simulink model "arabaStm"  (R2023b)
settings: Solver=FixedStepAuto  StartTime=0.0  StopTime=45  RelTol=1e-3  EnableMultiTasking=on
undefined symbols (not defined in the file): PosCtrlSpeedLimit
libraries: stm32f4xxblockslib x11, stm32blockslib x4, mcbpositiondecoderlib x3, simulink x1, lidarlib x1, slpidlib x1, mcbcontrolslib x1, slrealtimeiplib x1
settings Model: Creator=The MathWorks, Inc.  LastModifiedBy=yigit
settings OptimizationCC: EnhancedBackFolding=on  PassReuseOutputArgsAs=Individual arguments  ZeroExternalMemoryAtStartup=off  ZeroInternalMemoryAtStartup=off  MaxStackSize=64  OptimizeBlockOrder=speed  DifferentSizesBufferReuse=on  OptimizationCustomize=off  EfficientTunableParamExpr=on
settings DebuggingCC: ParameterTunabilityLossMsg=error  UnconnectedInputMsg=warning  UnconnectedOutputMsg=warning  UnconnectedLineMsg=warning  SubsystemReferenceDiagnosticForUnitTest=warning
settings HardwareCC: ProdBitPerPointer=32  ProdBitPerSizeT=32  ProdBitPerPtrDiffT=32  ProdLargestAtomicInteger=Long  ProdLargestAtomicFloat=Double  ProdWordSize=32  ProdLongLongMode=on  ProdHWDeviceType=ARM Compatible->ARM Cortex
settings ModelReferenceCC: EnableRefExpFcnMdlSchedulingChecks=on
settings SFSimCC: MATLABDynamicMemAlloc=off
settings RTWCC: Description=Embedded Coder  SystemTargetFile=ert.tlc  HardwareBoard=STM32F4xx Based  TemplateMakefile=ert_default_tmf  Toolchain=GNU Tools for ARM Embedded Processors  DLArmComputeVersion=19.05
settings CodeAppCC: ForceParamTrailComments=on  IgnoreCustomStorageClasses=off  OperatorAnnotations=on  SimulinkDataObjDesc=on  SFDataObjDesc=on  InsertBlockDesc=on
settings ERTTargetCC: CodeReplacementLibrary=ARM Cortex-M  ExtModeTransport=3  ExtModeStaticAlloc=on  ExtModeStaticAllocSize=8000  ExtModeMexFile=ext_xcp  ExtModeIntrfLevel=Level2 - Open

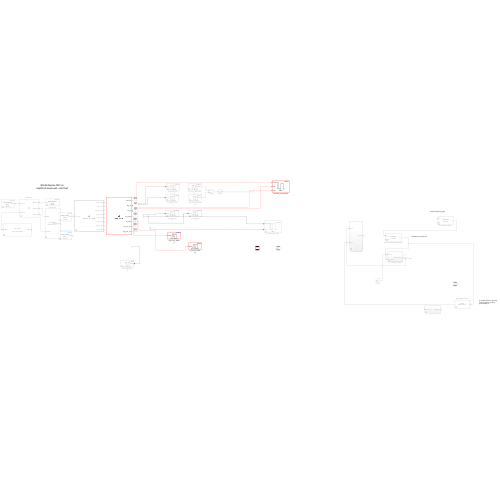
[thumbnail: Simulink's stored preview of the top-level diagram]
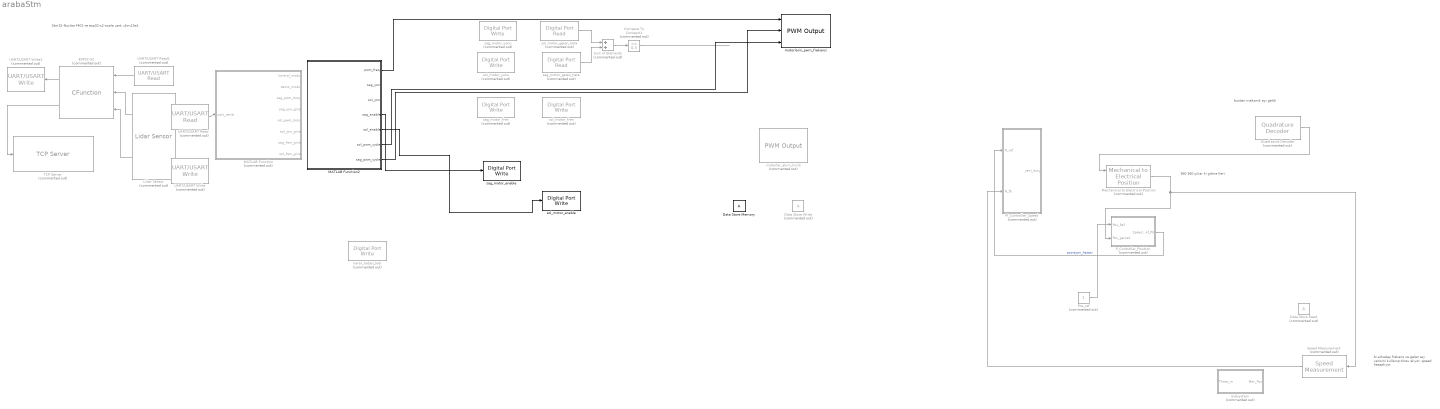
== system arabaStm ==
  note: bı arkadaş frekans ve gelen açı verisini kullanıp türev alıyor. speed hesaplıyor
  note: 360 360 çıkar ki gitme ileri.
  note: burdan mekanik açı geldi
  note: Stm32-Nucleo f401-re
      | esp32-s2-soala uart, uhm15a1
  Compare To Constant1 : simulink/Logic and Bit Operations/Compare To Constant  Commented=on  relop=>=  const=0.5  OutDataTypeStr=boolean
  Data Store Memory : DataStoreMemory  WriteAfterWriteMsg=warning  ShowAdditionalParam=off  OutDataTypeStr=single
  Data Store Read : DataStoreRead  Commented=on  IndexOptions=Index vector (dialog)  Indices=1  OutputSizes=1
  Data Store Write : DataStoreWrite  Commented=on  IndexOptions=Index vector (dialog)  Indices=1  OutputSizes=1
  ESP32-S2 : CFunction  Commented=on  StartCode=|
      | function [motor1_speed, motor2_speed, duration] = simulateESP32Block()
      | %#codegen
      | 
      | % Define the function to simulate ESP32 behavior
      | coder.inline('never');
      | coder.extrinsic('rand');
      | 
      | % Initialize the motor control data structure
      | data.motor1_speed = uint8(0);
      | data.motor2_speed = uint8(0);
      | data.duration = uint8(0);
      | 
      | % Call the function to simulate ESP32 behavior
      | data = simulateESP32();
      | 
      | % Extract the fields from the structure
      | motor1_speed = data.motor1_speed;
      | motor2_speed = data.motor2_speed;
      | duration = data.duration;
      | 
      | end
      | 
      | % Define the function simulateESP32 within the same file
      | function data = simulateESP32()
      | % Simulate receiving motor control data
      | 
      | % Initialize random seed
      | coder.extrinsic('rng');
      | rng('shuffle');
      | 
      | % Create a structure for motor control data
      | data.motor1_speed = uint8(rand() * 255);
      | data.motor2_speed = uint8(rand() * 255);
      | data.duration = uint8(rand() * 60);
      | 
      | end
  Lidar Sensor : lidarlib/Lidar Sensor  Commented=on  SensorIndex=1  UpdateRate=0.1  SensorPosition=[0 0.2 0]  SensorOrientation=[0 0 0]  ActorProfilesVariableName=disable  HostID=1  MaxRange=120  AzimuthLimits=[-180 180]  AzimuthResolution=0.16  UseCustomElevationAngles=off  ElevationAngles=[-25 -15.6 -11.3 -8.8:0.9:-4 -4:0.32:1.6 3.3 4.6 7 10.3 15]  ElevationLimits=[-20 20]  ElevationResolution=1.25  HasNoise=on  RangeAccuracy=0.002  FogVisibility=1000  Rainrate=0  OutputIntensity=off  OutputClusters=off
  MATLAB Function : MATLAB Function  Commented=on  TreatAsAtomicUnit=on
  MATLAB Function2 : MATLAB Function  TreatAsAtomicUnit=on
  Mechanical to Electrical Position : mcbpositiondecoderlib/Mechanical to Electrical Position  Commented=on  PolePairsInputType=Specify via dialog  NrPP=4  selectedRange=Per unit  MechOfstInputType=Input port  mechOffsetIn=0  maxAngleIn=1  InputDataType=single  VariantSelect=floating-point
      settings: LibrarySourceBlock=mcblib/Sensor Decoders/Mechanical to Electrical Position
  PI_Controller_Speed : Subsystem  Commented=on
  P_Controller_Position : Subsystem  Commented=on
  Pos_ref : Constant  Commented=on  OutDataTypeStr=single  SampleTime=-1
  Quadrature Decoder : mcbpositiondecoderlib/Quadrature Decoder  Commented=on  EncoderSlitsPerRevolution=1000  EncoderCountsPerSlit=4  CounterSize=16 bits  ExternalIndexCount=on  PositionUnit=Radians  PositionDataType=single  ParameterInputType=off  CountsPerRevInverseDataType=single
      settings: LibrarySourceBlock=mcblib/Sensor Decoders/Quadrature Decoder
  Speed Measurement : mcbpositiondecoderlib/Speed Measurement  Commented=on  PositionUnit=Radians  PositionScalingDatatype=uint32  SpeedCalculationMode=Maximum application speed  SampleTimeAsync=100e-6  MaximumApplicationSpeed=1000  SpeedResolution=5e-6  DelayLength=299  MaximumMeasurableSpeed=1000  MeasurableSpeedResolution=4.6566e-07  SpeedUnit=RPM  PerUnitSpeed=1000  SpeedDataType=single
      settings: LibrarySourceBlock=mcblib/Sensor Decoders/Speed Measurement
  Subsystem : Subsystem  Commented=on
  Sum of Elements : Sum  Commented=on  OutMin=2
  TCP Server : slrealtimeiplib/TCP Server  Priority=-1  Commented=on  useHostTargetConn=off  serverAddress=192.168.1.95  serverPort=8001
  UART/USART Read : stm32blockslib/UART//USART Read  Priority=2  Commented=on  UARTModule=USART6  DataType=uint8  DataLength=8  BlockingMode=off  BlockingTimeout=0.1  OutputLength=off  OutputStatus=off  SampleTime=-1
      settings: LibrarySourceBlock=stm32f4xxblockslib/UART//USART Read
  UART/USART Read1 : stm32blockslib/UART//USART Read  Priority=2  Commented=on  UARTModule=USART2  DataType=uint8  DataLength=8  BlockingMode=off  BlockingTimeout=0.1  OutputLength=off  OutputStatus=off  SampleTime=-1
      settings: LibrarySourceBlock=stm32f4xxblockslib/UART//USART Read
  UART/USART Write : stm32blockslib/UART//USART Write  Priority=1  Commented=on  UARTModule=USART6  LengthOfDataToSend=off  BlockingMode=off  BlockingTimeout=0.1  OutputStatus=off
      settings: LibrarySourceBlock=stm32f4xxblockslib/UART//USART Write
  UART/USART Write1 : stm32blockslib/UART//USART Write  Priority=1  Commented=on  UARTModule=USART1  LengthOfDataToSend=off  BlockingMode=off  BlockingTimeout=0.1  OutputStatus=off
      settings: LibrarySourceBlock=stm32f4xxblockslib/UART//USART Write
  karar_hatasi_ledi : stm32f4xxblockslib/Digital Port Write  Commented=on  PortName=GPIOB  PinNumber=[0]  ReadOperation=off  IOAsArray=on  EnableSimPort=off
      settings: AttributesFormatString=%<PinNumber>
  motorlar_akim_limiti : stm32f4xxblockslib/PWM Output  Commented=on  TimerModule=TIM3  DutycycleUnits=Percentage  EnableChannel1=on  EnableChannel2=off  EnableChannel3=off  EnableChannel4=off  EnableCounterInput=off  EnableMainOutputInput=off  EnableFrequencyInput=on  SetRCAfterCE=off  OutputDirection=off  OutputMainOutputEnableStatus=off  SampleTime=0.1  EnableSimPort=off  EnableUpdateEvent=off  EnableCaptureCompare1Event=off  EnableCaptureCompare2Event=off  EnableCaptureCompare3Event=off  EnableCaptureCompare4Event=off  EnableTriggerEvent=off  EnableBreakEvent=on  ProcessorFamily=STM32F4  hoistedMaskSrc=ECSoC/ECSimCodegen/PWM Output
  motorlarin_pwm_frekansi : stm32f4xxblockslib/PWM Output  TimerModule=TIM3  DutycycleUnits=Percentage  EnableChannel1=on  EnableChannel2=on  EnableChannel3=off  EnableChannel4=off  EnableCounterInput=off  EnableMainOutputInput=off  EnableFrequencyInput=on  SetRCAfterCE=off  OutputDirection=off  OutputMainOutputEnableStatus=off  SampleTime=0.1  EnableSimPort=off  EnableUpdateEvent=off  EnableCaptureCompare1Event=off  EnableCaptureCompare2Event=off  EnableCaptureCompare3Event=off  EnableCaptureCompare4Event=off  EnableTriggerEvent=off  EnableBreakEvent=on  ProcessorFamily=STM32F4  hoistedMaskSrc=ECSoC/ECSimCodegen/PWM Output
  sag_motor_enable : stm32f4xxblockslib/Digital Port Write  PortName=GPIOA  PinNumber=[7]  ReadOperation=off  IOAsArray=on  EnableSimPort=off
      settings: AttributesFormatString=%<PinNumber>
  sag_motor_fren : stm32f4xxblockslib/Digital Port Write  Commented=on  PortName=GPIOB  PinNumber=[1]  ReadOperation=off  IOAsArray=on  EnableSimPort=off
      settings: AttributesFormatString=%<PinNumber>
  sag_motor_gelen_hata : stm32f4xxblockslib/Digital Port Read  Commented=on  PortName=GPIOA  PinNumber=[10]  ReadOperation=on  IOAsArray=on  SampleTime=-1  EnableSimPort=off
      settings: AttributesFormatString=%<PinNumber>
  sag_motor_yonu : stm32f4xxblockslib/Digital Port Write  Commented=on  PortName=GPIOA  PinNumber=[0]  ReadOperation=off  IOAsArray=on  EnableSimPort=off
      settings: AttributesFormatString=%<PinNumber>
  sol_motor_enable : stm32f4xxblockslib/Digital Port Write  PortName=GPIOA  PinNumber=[10]  ReadOperation=off  IOAsArray=on  EnableSimPort=off
      settings: AttributesFormatString=%<PinNumber>
  sol_motor_fren : stm32f4xxblockslib/Digital Port Write  Commented=on  PortName=GPIOB  PinNumber=[2]  ReadOperation=off  IOAsArray=on  EnableSimPort=off
      settings: AttributesFormatString=%<PinNumber>
  sol_motor_gelen_hata : stm32f4xxblockslib/Digital Port Read  Commented=on  PortName=GPIOA  PinNumber=[11]  ReadOperation=on  IOAsArray=on  SampleTime=-1  EnableSimPort=off
      settings: AttributesFormatString=%<PinNumber>
  sol_motor_yonu : stm32f4xxblockslib/Digital Port Write  Commented=on  PortName=GPIOA  PinNumber=[1]  ReadOperation=off  IOAsArray=on  EnableSimPort=off
      settings: AttributesFormatString=%<PinNumber>
  wires:
  UART/USART Read/1 -> MATLAB Function/1(uart_verisi)
  UART/USART Read1/1 -> ESP32-S2/1
  ESP32-S2/1 -> UART/USART Write1/1
  ESP32-S2/2 -> TCP Server/1
  Lidar Sensor/1 -> ESP32-S2/2
  Lidar Sensor/2 -> ESP32-S2/3
  ? -> sag_motor_yonu/1
  Sum of Elements/1 -> Compare To Constant1/1
  Compare To Constant1/1 -> ?
  ? -> sol_motor_yonu/1
  ? -> sol_motor_fren/1
  ? -> sag_motor_fren/1
  ? -> karar_hatasi_ledi/1
  sol_motor_gelen_hata/1 -> Sum of Elements/1
  sag_motor_gelen_hata/1 -> Sum of Elements/2
  MATLAB Function2/1(pwm_freq) -> motorlarin_pwm_frekansi/1
  MATLAB Function2/7(sag_pwm_cycle) -> motorlarin_pwm_frekansi/2
  MATLAB Function2/6(sol_pwm_cycle) -> motorlarin_pwm_frekansi/3
  ? -> motorlar_akim_limiti/1
  ? -> motorlar_akim_limiti/2
  MATLAB Function2/4(sag_enable) -> sag_motor_enable/1
  MATLAB Function2/5(sol_enable) -> sol_motor_enable/1
  Quadrature Decoder/1 -> Mechanical to Electrical Position/1
  Mechanical to Electrical Position/1 -> P_Controller_Position/2(Pos_gercek), Speed Measurement/1
  P_Controller_Position/1(Speed_Ref_PU) -> PI_Controller_Speed/1(N_ref)  "pozisyon_hatasi"
  Speed Measurement/1 -> PI_Controller_Speed/2(N_fb)
  Pos_ref/1 -> P_Controller_Position/1(Pos_Ref)

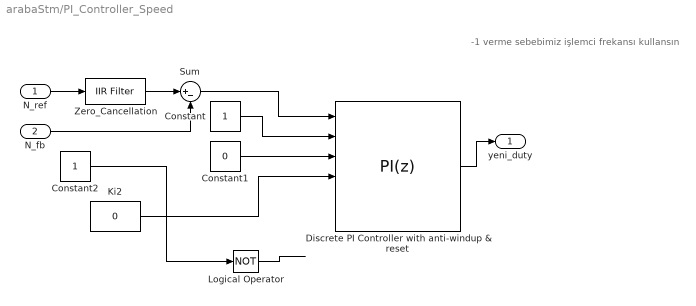
== system arabaStm/PI_Controller_Speed ==
  note: -1 verme sebebimiz işlemci frekansı kullansın
  N_ref : Inport
  N_fb : Inport  Port=2
  Constant : Constant
  Constant1 : Constant  Value=0
  Constant2 : Constant
  Discrete PI Controller with anti-windup & reset : slpidlib/PID Controller  Controller=PI  Form=Parallel  TimeDomain=Discrete-time  UseExternalTs=off  SampleTime=-1  IntegratorMethod=Forward Euler  FilterMethod=Forward Euler  ControllerParametersSource=external  P=1  I=1  UseKiTs=on  D=0  N=100  UseFilter=on  TunerSelectOption=Transfer Function Based (PID Tuner App)  InitialConditionSource=external  InitialConditionForIntegrator=0  InitialConditionForFilter=0  DifferentiatorICPrevScaledInput=0  ExternalReset=none  TrackingMode=off  Kt=1  LimitOutput=on  SatLimitsSource=external  UpperSaturationLimit=1  LowerSaturationLimit=-1  LinearizeAsGain=on  AntiWindupMode=none  Kb=1  LimitIntegrator=off  UpperIntegratorSaturationLimit=inf  LowerIntegratorSaturationLimit=-inf  RndMeth=Simplest  POutMin=[]  POutMax=[]  IOutMin=[]  IOutMax=[]  DOutMin=[]  DOutMax=[]  NOutMin=[]  NOutMax=[]  SumOutMin=[]  SumOutMax=[]  SaturationOutDataTypeStr=Inherit: Inherit via back propagation  SaturationOutMin=[]  SaturationOutMax=[]  PParamMin=[]  PParamMax=[]  IParamMin=[]  IParamMax=[]  DParamMin=[]  DParamMax=[]  NParamMin=[]  NParamMax=[]  KbParamMin=[]  KbParamMax=[]  KtParamMin=[]  KtParamMax=[]  KbOutMin=[]  KbOutMax=[]  KtOutMin=[]  KtOutMax=[]  IntegratorOutMin=[]  IntegratorOutMax=[]  FilterOutMin=[]  FilterOutMax=[]  SumI1OutMin=[]  SumI1OutMax=[]  SumI2OutMin=[]  SumI2OutMax=[]  SumI3OutMin=[]  SumI3OutMax=[]  SumI4OutMin=[]  SumI4OutMax=[]  SumDOutMin=[]  SumDOutMax=[]  DifferentiatorOutMin=[]  DifferentiatorOutMax=[]  FilterDiffOutCoefMin=[]  FilterDiffOutCoefMax=[]  ReciprocalOutMin=[]  ReciprocalOutMax=[]  SumDenOutMin=[]  SumDenOutMax=[]  SumNumOutMin=[]  SumNumOutMax=[]  DivideOutMin=[]  DivideOutMax=[]  UdiffTsProdOutMin=[]  UdiffTsProdOutMax=[]  NTsProdOutMin=[]  NTsProdOutMax=[]  UintegralTsProdOutMin=[]  UintegralTsProdOutMax=[]  UngainTsProdOutMin=[]  UngainTsProdOutMax=[]  ClampingZeroOutDataTypeStr=Inherit: Inherit via back propagation  ClampingZeroOutMin=[]  ClampingZeroOutMax=[]  FilterDenConstantOutDataTypeStr=Inherit: Inherit via back propagation  FilterDenConstantOutMin=[]  FilterDenConstantOutMax=[]  PCopyOutDataTypeStr=Inherit: Inherit via back propagation  PCopyOutMin=[]  PCopyOutMax=[]  NCopyOutDataTypeStr=Inherit: Inherit via back propagation  NCopyOutMin=[]  NCopyOutMax=[]  IntegratorContinuousStateAttributes=''  IntegratorStateMustResolveToSignalObject=off  IntegratorRTWStateStorageClass=Auto  FilterContinuousStateAttributes=''  FilterStateMustResolveToSignalObject=off  FilterRTWStateStorageClass=Auto  ParallelPVariant=ExternalParameters  IdealPVariant=Disabled  IVariant=ExternalParameters  DVariant=Disabled  IntegratorVariant=Discrete  SatVariant=External  AWVariant=Passthrough  PCopyVariant=Disabled  TRVariant=Disabled  FdbkBlocksVariant=Forward  IdealPFdbkVariant=Disabled  SatFdbkVariant=Disabled  DerivativeFilterVariant=Disabled  NVariant=Disabled  NCopyVariant=Disabled_SignalSpec  FilterICVariant=Disabled  IntegratorICVariant=ExternalICs  ExternalResetVariant=Disabled  TRSumVariant=Passthrough  SumFdbkVariant=Disabled  SumVariant=Sum_PI  TsampFilterVariant=InternalTs  TsampNgainVariant=Passthrough  TsampIntegralVariant=Disabled_SignalSpec  ExternalSaturationOutDataTypeStr=Inherit: Same as second input
      settings: LibrarySourceBlock=mcbcontrolslib/PI Controller
  Ki2 : Constant  Value=0  OutDataTypeStr=single  SampleTime=-1
  Logical Operator : Logic  Operator=NOT  IconShape=distinctive  AllPortsSameDT=off  OutDataTypeStr=boolean
  Sum : Sum  Inputs=|+-  RndMeth=Round
  Zero_Cancellation : mcbcontrolslib/IIR Filter  VariantControl=Low Pass Filter  VariantSelect=Low-pass  Filter_constant=0.01  advancedSettings=off  Ts=50e-6  cutOff_freq=32.1525
  yeni_duty : Outport  VectorParamsAs1DForOutWhenUnconnected=off
  wires:
  Discrete PI Controller with anti-windup & reset/1 -> yeni_duty/1
  Constant1/1 -> Discrete PI Controller with anti-windup & reset/3
  Constant/1 -> Discrete PI Controller with anti-windup & reset/2
  N_fb/1 -> Sum/2
  N_ref/1 -> Zero_Cancellation/1
  Logical Operator/1 -> ?
  Ki2/1 -> Discrete PI Controller with anti-windup & reset/4
  Sum/1 -> Discrete PI Controller with anti-windup & reset/1
  Constant2/1 -> Logical Operator/1
  Zero_Cancellation/1 -> Sum/1

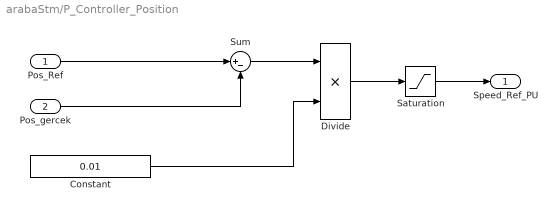
== system arabaStm/P_Controller_Position ==
  Pos_Ref : Inport
  Pos_gercek : Inport  Port=2
  Constant : Constant  Value=0.01  OutDataTypeStr=single  SampleTime=-1
  Divide : Product  Inputs=**  OutDataTypeStr=single  RndMeth=Simplest
  Saturation : Saturate  UpperLimit=PosCtrlSpeedLimit  LowerLimit=-PosCtrlSpeedLimit
  Sum : Sum  Inputs=|+-  OutDataTypeStr=Inherit: Same as first input
  Speed_Ref_PU : Outport
  wires:
  Constant/1 -> Divide/2
  Saturation/1 -> Speed_Ref_PU/1
  Divide/1 -> Saturation/1
  Pos_Ref/1 -> Sum/1
  Pos_gercek/1 -> Sum/2
  Sum/1 -> Divide/1

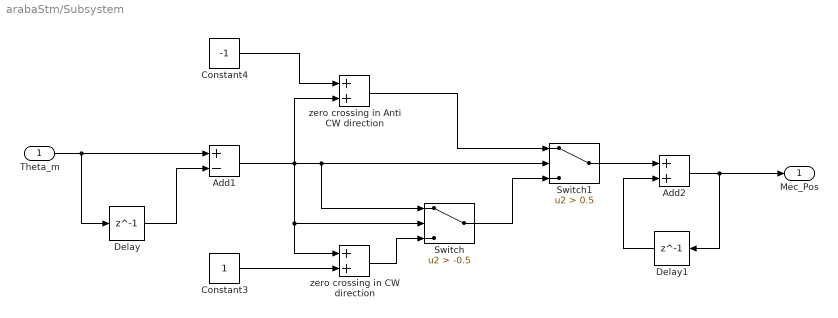
== system arabaStm/Subsystem ==
  Theta_m : Inport
  Add1 : Sum  Inputs=+-
  Add2 : Sum
  Constant3 : Constant  OutDataTypeStr=dataType
  Constant4 : Constant  Value=-1  OutDataTypeStr=dataType
  Delay : Delay  DelayLength=1
  Delay1 : Delay  DelayLength=1
  Switch : Switch  Criteria=u2 > Threshold  Threshold=-0.5  SaturateOnIntegerOverflow=off  InputSameDT=off
  Switch1 : Switch  Criteria=u2 > Threshold  Threshold=0.5  SaturateOnIntegerOverflow=off  InputSameDT=off
  zero crossing in Anti CW direction : Sum
  zero crossing in CW direction : Sum
  Mec_Pos : Outport
  wires:
  Theta_m/1 -> Delay/1, Add1/1
  Switch1/1 -> Add2/1
  Delay/1 -> Add1/2
  Add1/1 -> zero crossing in Anti CW direction/2, zero crossing in CW direction/1, Switch/2, Switch/1, Switch1/2
  Switch/1 -> Switch1/3
  Constant3/1 -> zero crossing in CW direction/2
  Add2/1 -> Mec_Pos/1, Delay1/1
  zero crossing in Anti CW direction/1 -> Switch1/1
  Delay1/1 -> Add2/2
  Constant4/1 -> zero crossing in Anti CW direction/1
  zero crossing in CW direction/1 -> Switch/3

== matlab function arabaStm/MATLAB Function ==
  data: uart_verisi input; kontrol_modu output; demo_modu output; sag_pwm_duty output; sag_yon_giris output; sol_pwm_duty output; sol_yon_giris output; sag_fren_giris output; sol_fren_giris output
function [kontrol_modu, demo_modu, sag_pwm_duty, sag_yon_giris, sol_pwm_duty, sol_yon_giris, sag_fren_giris, sol_fren_giris] = process_uart_data(uart_verisi)
    % UART verisini işleyerek kontrol sinyallerini çıkartır
    % Başlık çıkarma
    baslik = uart_verisi(1);
    
    % Varsayılan değerler
    kontrol_modu = uint8(2); % Başlangıç değeri olarak demo modu
    demo_modu = uint8(1); % Demo modu 1 seçeneği başlangıç olarak
    sag_pwm_duty = 0.0; % PWM duty cycle başlangıç olarak 0.0
    sag_yon_giris = uint8(0);
    sol_pwm_duty = 0.0; % PWM duty cycle başlangıç olarak 0.0
    sol_yon_giris = uint8(0);
    sag_fren_giris = uint8(0);
    sol_fren_giris = uint8(0);
    
    if baslik ~= 0xAA
        % Geçersiz başlık, varsayılan demo modu 1'i seç
        return;
    end
    
    % Kontrol modu, demo modu ve veriyi çıkarma
    kontrol_modu = uart_verisi(2);
    demo_modu = uart_verisi(3);
    kontrol_verisi = uart_verisi(4:7);  % Gerekli veri uzunluğuna göre ayarlandı
    fren_verisi = uart_verisi(8:9);     % Gerekli veri uzunluğuna göre ayarlandı
    
    % Kontrol verilerini değişkenlere atama
    sag_pwm_duty = double(kontrol_verisi(1)) / 255.0; % 0-255 arası değeri 0.0-1.0 arasına çevir
    sag_yon_giris = kontrol_verisi(2);
    sol_pwm_duty = double(kontrol_verisi(3)) / 255.0; % 0-255 arası değeri 0.0-1.0 arasına çevir
    sol_yon_giris = kontrol_verisi(4);
    sag_fren_giris = fren_verisi(1);
    sol_fren_giris = fren_verisi(2);
end

== matlab function arabaStm/MATLAB Function2 ==
  data: pwm_freq output; sag_yon output; sol_yon output; sag_enable output; sol_enable output; sol_pwm_cycle output; sag_pwm_cycle output
function [pwm_freq, sag_yon, sol_yon, sag_enable, sol_enable, sol_pwm_cycle, sag_pwm_cycle] = motor_secici
%#codegen

% Sabit PWM frekansı
pwm_freq = uint32(13500);  % 13.5 kHz

% Başlangıç değerlerini ayarla
sag_pwm_cycle = uint8(0);  % Sağ motor PWM duty cycle (0.0 to 1.0)
sag_yon = uint8(0);   % Sağ motor yön kontrolü
sol_pwm_cycle = uint8(0);  % Sol motor PWM duty cycle (0.0 to 1.0)
sol_yon = uint8(0);   % Sol motor yön kontrolü
sag_enable = uint8(0);  % Sağ motor enable sinyali
sol_enable = uint8(0);  % Sol motor enable sinyali

% Demo modud
if true
    sag_enable = uint8(1);
    sol_enable = uint8(1);
    sag_pwm_cycle = uint8(80); % %80 duty cycle
    sol_pwm_cycle = uint8(30); % %70 duty cycle
    
    % Burada gecikmeyi STM32F4 için zamanlayıcı (timer) kullanarak sağlamak gerekir
    % Örneğin: HAL_Delay(1000); % 1 saniye bekle
end

end
